simulink model "rlsGradientEst_th"  (R2022a)
settings: Solver=FixedStepAuto  StartTime=0.0  StopTime=duration  FixedStep=1  RelTol=1e-3
libraries: rlsGradientEst_cl x1
settings Model: Creator=mcobb  LastModifiedBy=lhill8
settings SolverCC: AlgebraicLoopSolver=TrustRegion
settings DebuggingCC: UnconnectedInputMsg=warning  UnconnectedOutputMsg=warning  UnconnectedLineMsg=warning  SFMachineParentedDataDiag=warning  ArithmeticOperatorsInVariantConditions=warning
settings SFSimCC: CustomCodeUndefinedFunction=UseInterfaceOnly

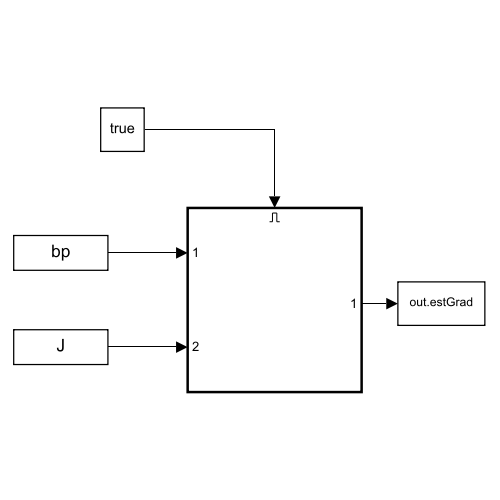
[thumbnail: Simulink's stored preview of the top-level diagram]
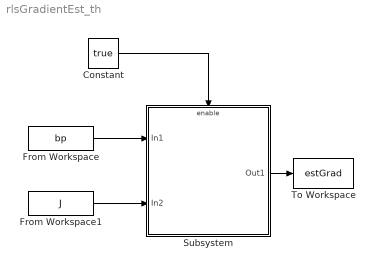
== system rlsGradientEst_th ==
  Constant : Constant  Value=true
  From Workspace : FromWorkspace  VariableName=bp
  From Workspace1 : FromWorkspace  VariableName=J
  Subsystem : Subsystem
  To Workspace : ToWorkspace  VariableName=estGrad  SaveFormat=Timeseries  SampleTime=-1
  wires:
  From Workspace/1 -> Subsystem/1(In1)
  From Workspace1/1 -> Subsystem/2(In2)
  Subsystem/1(Out1) -> To Workspace/1
  Constant/1 -> Subsystem/Enable

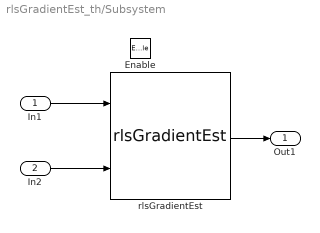
== system rlsGradientEst_th/Subsystem ==
  In1 : Inport
  In2 : Inport  Port=2
  Enable : EnablePort
  rlsGradientEst : rlsGradientEst_cl/rlsGradientEst  AdaptationParameter=AdaptationParameter  Ts=1  numParams=1
  Out1 : Outport  VectorParamsAs1DForOutWhenUnconnected=off
  wires:
  In2/1 -> rlsGradientEst/2
  rlsGradientEst/1 -> Out1/1
  In1/1 -> rlsGradientEst/1
